simulink model "general_system"  (R2018a)
settings: Solver=FixedStepAuto  StartTime=0.0  StopTime=3.0  FixedStep=1e-6  RelTol=1e-3
undefined symbols (not defined in the file): A, B, opt_theorem, P, Q, sys, xe
settings Model: Creator=julio  LastModifiedBy=julio

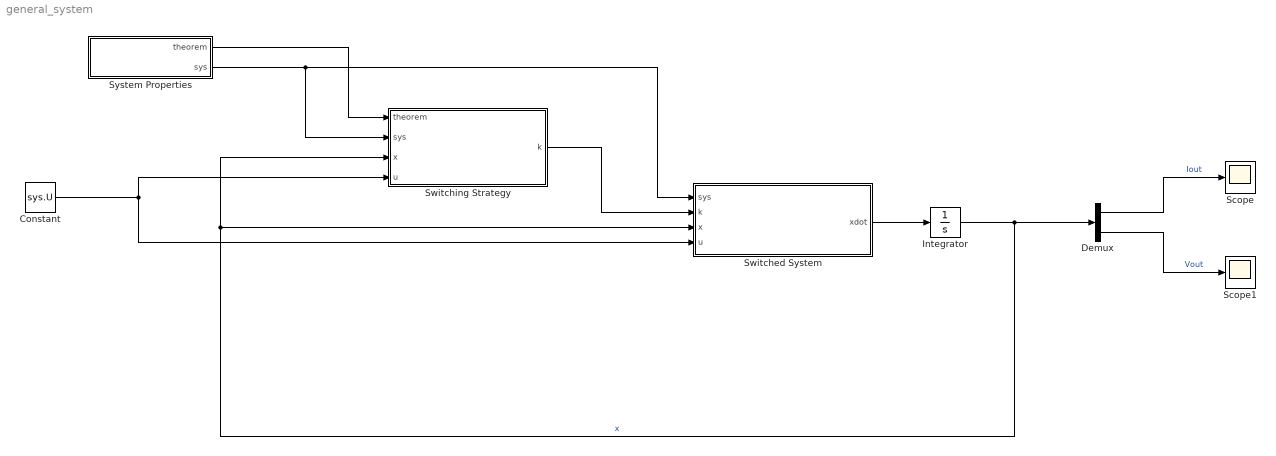
== system general_system ==
  Constant : Constant  Value=sys.U
  Demux : Demux  Outputs=2
  Integrator : Integrator  InitialCondition=sys.x0
  Scope : Scope
  Scope1 : Scope
  Switched System : MATLAB Function  TreatAsAtomicUnit=on
  Switching Strategy : MATLAB Function  TreatAsAtomicUnit=on
  System Properties : Subsystem
  wires:
  Switched System/1(xdot) -> Integrator/1
  Integrator/1 -> Switched System/3(x), Switching Strategy/3(x), Demux/1  "x"
  Constant/1 -> Switched System/4(u), Switching Strategy/4(u)
  System Properties/2(sys) -> Switched System/1(sys), Switching Strategy/2(sys)
  Switching Strategy/1(k) -> Switched System/2(k)
  System Properties/1(theorem) -> Switching Strategy/1(theorem)
  Demux/1 -> Scope/1  "Iout"
  Demux/2 -> Scope1/1  "Vout"

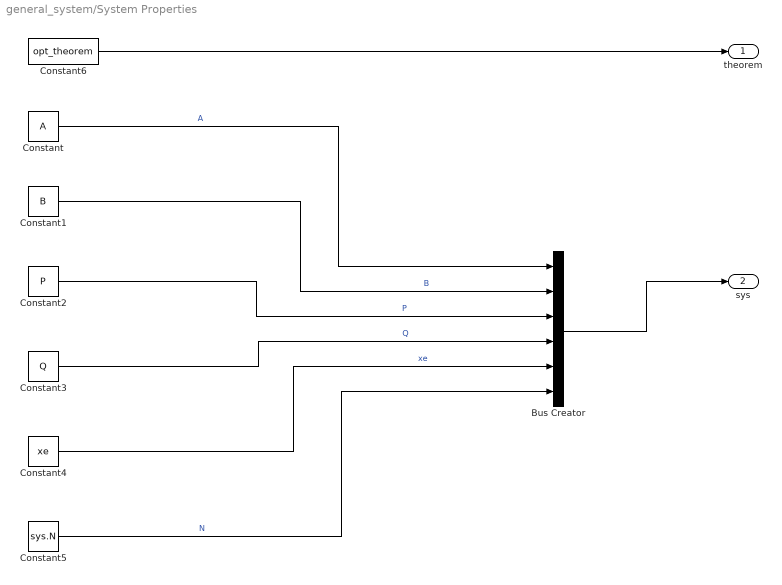
== system general_system/System Properties ==
  Bus Creator : BusCreator  Inputs=6  OutDataTypeStr=Bus: SystemDataBus
  Constant : Constant  Value=A  VectorParams1D=off
  Constant1 : Constant  Value=B  VectorParams1D=off
  Constant2 : Constant  Value=P  VectorParams1D=off
  Constant3 : Constant  Value=Q  VectorParams1D=off
  Constant4 : Constant  Value=xe  VectorParams1D=off
  Constant5 : Constant  Value=sys.N
  Constant6 : Constant  Value=opt_theorem
  theorem : Outport
  sys : Outport  Port=2
  wires:
  Bus Creator/1 -> sys/1
  Constant2/1 -> Bus Creator/3  "P"
  Constant1/1 -> Bus Creator/2  "B"
  Constant/1 -> Bus Creator/1  "A"
  Constant3/1 -> Bus Creator/4  "Q"
  Constant4/1 -> Bus Creator/5  "xe"
  Constant5/1 -> Bus Creator/6  "N"
  Constant6/1 -> theorem/1

== matlab function general_system/Switched System ==
  data: sys input; k input; x input; u input; xdot output
function xdot = switched_system(sys, k, x, u)
    xdot = sys.A(:,:,k)*x + sys.B(:,:,k)*u;
end

== matlab function general_system/Switching Strategy ==
  data: theorem input; sys input; x input; u input; k output
function k = switching_strategy(theorem, sys, x, u)
    qsi = x - sys.xe;
    sig = zeros(sys.N,1);
    
    for i=1:sys.N
        switch(theorem)
            case 1
                sig(i) = qsi'*(sys.Q(:,:,i)*qsi + 2*sys.P*(sys.A(:,:,i)*x + sys.B(:,:,i)*u));
            case 2
                sig(i) = qsi'*sys.P*(sys.A(:,:,i)*sys.xe + sys.B(:,:,i)*u);
        end
    end
    [~, k] = min(sig);
end
